simulink model "auto"  (Simulink 7.6)
settings: Solver=ode45  StartTime=0.0  StopTime=60  RelTol=1e-3
settings Model: Creator=Bogdy  LastModifiedBy=Bogdy

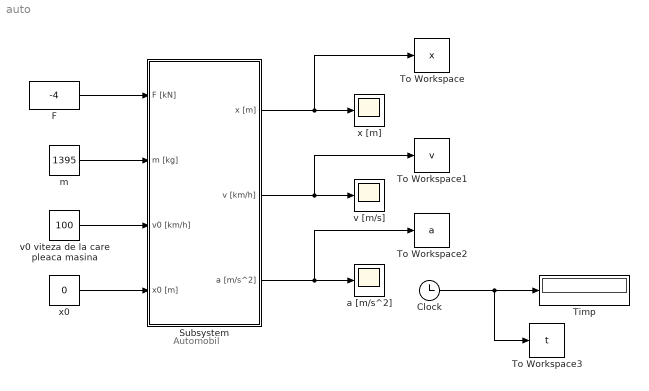
== system auto ==
  note: Automobil
  Clock : Clock
      settings: Decimation=10
  F : Constant  Value=-4
  Subsystem : Subsystem
  Timp : Display
  To Workspace : ToWorkspace  VariableName=x  SampleTime=-1  SaveFormat=Array
  To Workspace1 : ToWorkspace  VariableName=v  SampleTime=-1  SaveFormat=Array
  To Workspace2 : ToWorkspace  VariableName=a  SampleTime=-1  SaveFormat=Array
  To Workspace3 : ToWorkspace  VariableName=t  SampleTime=-1  SaveFormat=Array
  a [m/s^2] : Scope
      settings: SaveName=ScopeData2
  m : Constant  Value=1395
  "v [m/s] " : Scope
      settings: TimeRange=60  YMin=0  YMax=2500000
  v0 viteza de la care pleaca masina : Constant  Value=100
  x [m] : Scope
  x0 : Constant  Value=0
  wires:
  F/1 -> Subsystem/1(F [kN])
  m/1 -> Subsystem/2(m [kg])
  v0 viteza de la care pleaca masina/1 -> Subsystem/3(v0 [km/h])
  x0/1 -> Subsystem/4(x0 [m])
  Subsystem/1(x [m]) -> x [m]/1, To Workspace/1
  Subsystem/2(v [km/h]) -> To Workspace1/1, "v [m/s] "/1
  Subsystem/3(a [m/s^2]) -> a [m/s^2]/1, To Workspace2/1
  Clock/1 -> Timp/1, To Workspace3/1

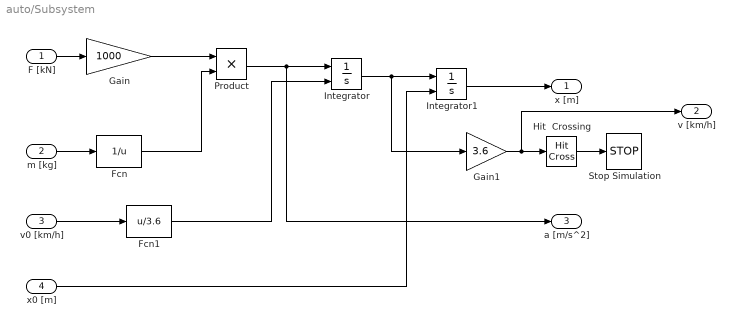
== system auto/Subsystem ==
  F [kN] : Inport
  m [kg] : Inport  Port=2
  v0 [km/h] : Inport  Port=3
  x0 [m] : Inport  Port=4
  Fcn : Fcn  Expr=1/u
  Fcn1 : Fcn  Expr=u/3.6
  Gain : Gain  Gain=1000
  Gain1 : Gain  Gain=3.6
  Hit  Crossing : HitCross  HitCrossingDirection=falling
  Integrator : Integrator  InitialConditionSource=external
  Integrator1 : Integrator  InitialConditionSource=external
  Product : Product  RndMeth=Zero
  Stop Simulation : Stop
  x [m] : Outport
  v [km/h] : Outport  Port=2
  a [m/s^2] : Outport  Port=3
  wires:
  F [kN]/1 -> Gain/1
  Product/1 -> a [m/s^2]/1, Integrator/1
  m [kg]/1 -> Fcn/1
  Fcn/1 -> Product/2
  v0 [km/h]/1 -> Fcn1/1
  Fcn1/1 -> Integrator/2
  Integrator/1 -> Integrator1/1, Gain1/1
  Integrator1/1 -> x [m]/1
  x0 [m]/1 -> Integrator1/2
  Gain/1 -> Product/1
  Gain1/1 -> Hit  Crossing/1, v [km/h]/1
  Hit  Crossing/1 -> Stop Simulation/1
